simulink model "maxpid_frottements_visqueux"  (Simulink 7.3)
settings: Solver=ode3  StartTime=0.0  StopTime=1  FixedStep=1e-3  RelTol=1e-3
settings Model: Creator=Renaud MERLE  LastModifiedBy=Renaud MERLE

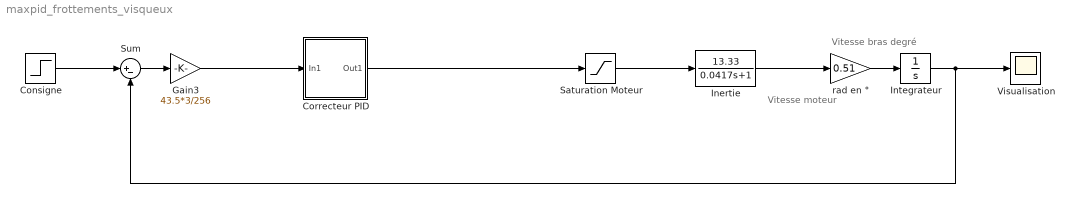
== system maxpid_frottements_visqueux ==
  note: Vitesse
      | moteur
  note: Vitesse
      | bras degré
  Consigne : Step  Time=0  After=30  SampleTime=0
  Correcteur PID : Subsystem
  Gain3 : Gain  Gain=43.5*3/256  ParameterDataType=fixdt(1, 16)  ParameterScaling=2^0  OutDataType=fixdt(1, 16)  OutScaling=2^0
  Inertie : TransferFcn  Numerator=[13.33]  Denominator=[0.0417 1]
  Integrateur : Integrator
  Saturation Moteur : Saturate  UpperLimit=25  LowerLimit=-25  OutDataType=fixdt(1, 16)  OutScaling=2^0
  Sum : Sum  Inputs=|+-  OutDataType=fixdt(1, 16)  OutScaling=2^0
  Visualisation : Scope
  rad en ° : Gain  Gain=0.51  ParameterDataType=fixdt(1, 16)  ParameterScaling=2^0  OutDataType=fixdt(1, 16)  OutScaling=2^0
  wires:
  Consigne/1 -> Sum/1
  Sum/1 -> Gain3/1
  rad en °/1 -> Integrateur/1
  Integrateur/1 -> Sum/2, Visualisation/1
  Correcteur PID/1(Out1) -> Saturation Moteur/1
  Saturation Moteur/1 -> Inertie/1
  Inertie/1 -> rad en °/1
  Gain3/1 -> Correcteur PID/1(In1)

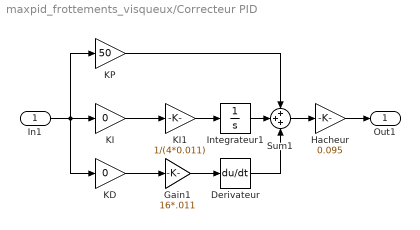
== system maxpid_frottements_visqueux/Correcteur PID ==
  In1 : Inport
  Derivateur : Derivative
  Gain1 : Gain  Gain=16*.011  ParameterDataType=fixdt(1, 16)  ParameterScaling=2^0  OutDataType=fixdt(1, 16)  OutScaling=2^0
  Hacheur : Gain  Gain=0.095  ParameterDataType=fixdt(1, 16)  ParameterScaling=2^0  OutDataType=fixdt(1, 16)  OutScaling=2^0
  Integrateur1 : Integrator
  KD : Gain  Gain=0  ParameterDataType=fixdt(1, 16)  ParameterScaling=2^0  OutDataType=fixdt(1, 16)  OutScaling=2^0
  KI : Gain  Gain=0  ParameterDataType=fixdt(1, 16)  ParameterScaling=2^0  OutDataType=fixdt(1, 16)  OutScaling=2^0
  KI1 : Gain  Gain=1/(4*0.011)  ParameterDataType=fixdt(1, 16)  ParameterScaling=2^0  OutDataType=fixdt(1, 16)  OutScaling=2^0
  KP : Gain  Gain=50  ParameterDataType=fixdt(1, 16)  ParameterScaling=2^0  OutDataType=fixdt(1, 16)  OutScaling=2^0
  Sum1 : Sum  Inputs=+++  OutDataType=fixdt(1, 16)  OutScaling=2^0
  Out1 : Outport
  wires:
  In1/1 -> KD/1, KP/1, KI/1
  KP/1 -> Sum1/1
  KI/1 -> KI1/1
  KD/1 -> Gain1/1
  Integrateur1/1 -> Sum1/2
  Derivateur/1 -> Sum1/3
  Sum1/1 -> Hacheur/1
  Gain1/1 -> Derivateur/1
  KI1/1 -> Integrateur1/1
  Hacheur/1 -> Out1/1
